simulink model "IGM_2D_SP"  (R2021a)
settings: Solver=VariableStepAuto  StartTime=0.0  StopTime=1000  RelTol=1e-3
values from neighbouring files (symbols this model uses):
  X0 = [x0;y0;vx0;vy0]    [Main.m]
undefined symbols (not defined in the file or in its folder): p
settings Model: Creator=FawadFarooq  LastModifiedBy=FawadFarooq

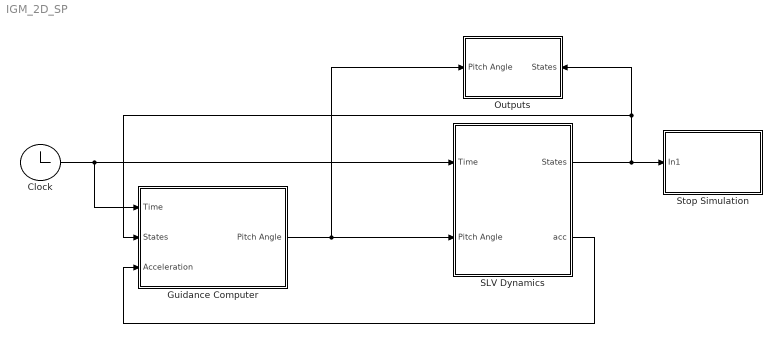
== system IGM_2D_SP ==
  Clock : Clock
  Guidance Computer : Subsystem
  Outputs : Subsystem
      settings: PortSchema="{\"entries\":[{\"content\":{\"sides\":[{\"content\":{\"connectorIds\":[\"In1\"]},\"type\":\"ConnectorPlacement.EquallySpacedRectSide\",\"uuid\":\"072ea4b5-769e-43eb-a3c3-6af6f3856208\"},{\"content\":{\"connectorIds\":[\"In2\"],\"side\":\"RIGHT\"},\"type\":\"ConnectorPlacement.EquallySpacedRectSide\",\"uuid\":\"64728ef0-65f2-4c87-b895-8041e6a7d13d\"},{\"content\":{\"connectorIds\":[],\"side\":\"TOP\"},\"type\":\"ConnectorPlacement.EquallySpacedRectSide\",\"uuid\":\"9708094a-022a-48f5-847a-dae2381fa515\"}]},\"type\":\"ConnectorPlacement.EquallySpacedConnector\",\"uuid\":\"193dd09d-2000-471e-91a9-709041d894d9\"}],\"packageUris\":[\"http://schema.mathworks.com/mf0/Connector/R2020b\"],\"version\":\"1.0\"}"
  SLV Dynamics : Subsystem
  Stop Simulation : Subsystem
  wires:
  Clock/1 -> SLV Dynamics/1(Time), Guidance Computer/1(Time)
  SLV Dynamics/1(States) -> Stop Simulation/1(In1), Outputs/2(States), Guidance Computer/2(States)
  Guidance Computer/1(Pitch Angle) -> Outputs/1(Pitch Angle), SLV Dynamics/2(Pitch Angle)
  SLV Dynamics/2(acc) -> Guidance Computer/3(Acceleration)

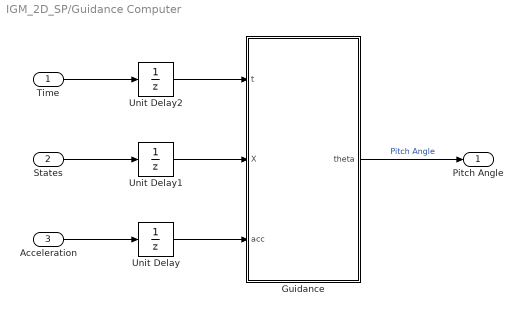
== system IGM_2D_SP/Guidance Computer ==
  Time : Inport
  States : Inport  Port=2
  Acceleration : Inport  Port=3
  Guidance : MATLAB Function  TreatAsAtomicUnit=on  SystemSampleTime=p.Tsamp
  Unit Delay : UnitDelay  InitialCondition=p.Thr/p.m0  SampleTime=-1  HasFrameUpgradeWarning=on
  Unit Delay1 : UnitDelay  InitialCondition=X0  SampleTime=-1  HasFrameUpgradeWarning=on
  Unit Delay2 : UnitDelay  InitialCondition=p.Tsamp  SampleTime=-1  HasFrameUpgradeWarning=on
  Pitch Angle : Outport
  wires:
  Guidance/1(theta) -> Pitch Angle/1  "Pitch Angle"
  Unit Delay2/1 -> Guidance/1(t)
  Unit Delay/1 -> Guidance/3(acc)
  Acceleration/1 -> Unit Delay/1
  Unit Delay1/1 -> Guidance/2(X)
  States/1 -> Unit Delay1/1
  Time/1 -> Unit Delay2/1

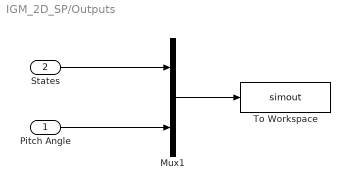
== system IGM_2D_SP/Outputs ==
  Pitch Angle : Inport
  States : Inport  Port=2
  Mux1 : Mux  Inputs=2
  To Workspace : ToWorkspace  VariableName=simout  SaveFormat=Timeseries  SampleTime=-1
  wires:
  States/1 -> Mux1/1
  Mux1/1 -> To Workspace/1
  Pitch Angle/1 -> Mux1/2

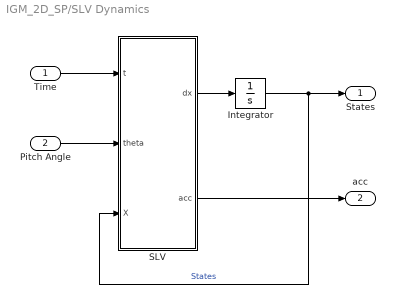
== system IGM_2D_SP/SLV Dynamics ==
  Time : Inport
  Pitch Angle : Inport  Port=2
  Integrator : Integrator  InitialCondition=X0
  SLV : MATLAB Function  TreatAsAtomicUnit=on
  States : Outport
  acc : Outport  Port=2
  wires:
  SLV/1(dx) -> Integrator/1
  Time/1 -> SLV/1(t)
  Integrator/1 -> States/1, SLV/3(X)  "States"
  Pitch Angle/1 -> SLV/2(theta)
  SLV/2(acc) -> acc/1

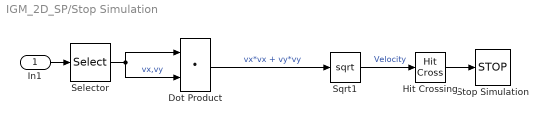
== system IGM_2D_SP/Stop Simulation ==
  In1 : Inport
  Dot Product : DotProduct  InputSameDT=on  OutDataTypeStr=Inherit: Inherit via internal rule
  Hit Crossing : HitCross  HitCrossingOffset=p.vf  HitCrossingDirection=rising
  Selector : Selector  InputPortWidth=4  IndexOptions=Index vector (dialog)  Indices=[3 4]  OutputSizes=1
  Sqrt1 : Sqrt  SaturateOnIntegerOverflow=on
  Stop Simulation : Stop
  wires:
  Hit Crossing/1 -> Stop Simulation/1
  In1/1 -> Selector/1
  Selector/1 -> Dot Product/2, Dot Product/1  "vx,vy"
  Dot Product/1 -> Sqrt1/1  "vx*vx + vy*vy"
  Sqrt1/1 -> Hit Crossing/1  "Velocity"

== matlab function IGM_2D_SP/Guidance Computer/Guidance ==
  settings: updateMethod=DISCRETE  sampleTime=0.02
  data: t input; theta output; X input; acc input; p parameter
function theta = fcn(t, X, acc, p) %#ok<*INUSL>

theta = igm_2d_sp(t, X, acc, p);

== matlab function IGM_2D_SP/SLV Dynamics/SLV ==
  data: t input; theta input; dx output; X input; acc output; p parameter
function [dx,acc] = fcn(t,theta,X,p)

u = [cosd(theta);
    sind(theta)];

mass = p.m0 - p.mdot*t;
acc = p.Thr/mass;

r = norm([X(1);X(2)]);

rdot = [X(3);
    X(4)];

vdot = acc*u - (p.GM/r^3)*[X(1);X(2)];

dx = [rdot;vdot];
